simulink model "W02_B_three_ways"  (R2024b)
settings: Solver=ode4  StartTime=0  StopTime=T_final  FixedStep=h  RelTol=1e-3
values from neighbouring files (symbols this model uses):
  F_step = 1    [W02_0_setup.m]
  pid_b = 2    [W02_0_setup.m]
  pid_k = 2    [W02_0_setup.m]
  pid_m = 1    [W02_0_setup.m]
  t_step = 1    [W02_0_setup.m]
  x0_pos = 0    [W02_0_setup.m]    (also in W02_1_build_pid.m = 0.5 and Run: A and C swing back from 0.5 m,',    'B stays at)
  x0_vel = 0    [W02_0_setup.m]
settings Model: Creator=admin  LastModifiedBy=admin
settings DataIOCC: ReturnWorkspaceOutputs=off

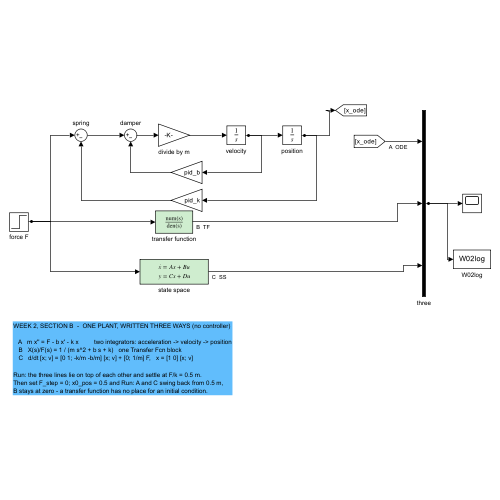
[thumbnail: Simulink's stored preview of the top-level diagram]
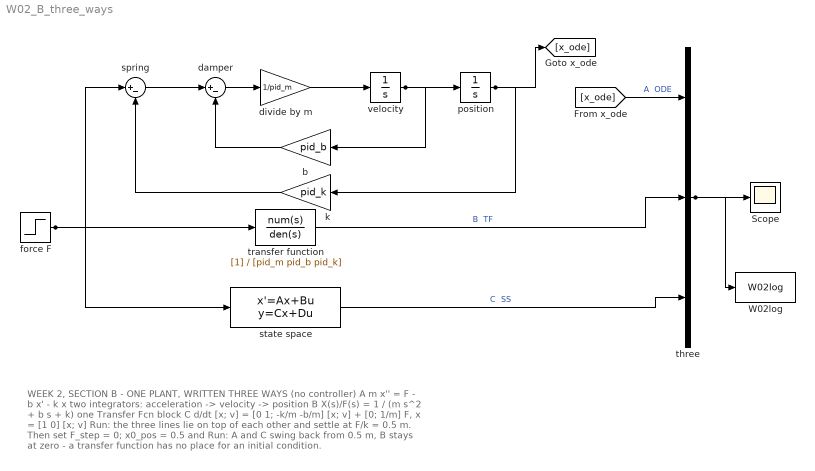
== system W02_B_three_ways ==
  note: WEEK 2, SECTION B  -  ONE PLANT, WRITTEN THREE WAYS (no controller)
      |
      |    A   m x'' = F - b x' - k x         two integrators: acceleration -> velocity -> position
      |    B   X(s)/F(s) = 1 / (m s^2 + b s + k)   one Transfer Fcn block
      |    C   d/dt [x; v] = [0 1; -k/m -b/m] [x; v] + [0; 1/m] F,   x = [1 0] [x; v]
      |
      | Run: the three lines lie on top of each other and settle at F/k = 0.5 m.
      | Then set F_step = 0; x0_pos = 0.5 and Run: A and C swing back from 0.5 m,
      | B stays at zero - a transfer function has no place for an initial condition.
  Scope : Scope
  W02log : ToWorkspace  VariableName=W02log  SaveFormat=Structure With Time  SampleTime=-1
  b : Gain  Gain=pid_b
  damper : Sum  Inputs=|+-
  divide by m : Gain  Gain=1/pid_m
  force F : Step  Time=t_step  After=F_step  SampleTime=0
  k : Gain  Gain=pid_k
  position : Integrator  InitialCondition=x0_pos
  spring : Sum  Inputs=|+-
  state space : StateSpace  A=[0 1; -pid_k/pid_m -pid_b/pid_m]  B=[0; 1/pid_m]  C=[1 0]  D=0  InitialCondition=[x0_pos; x0_vel]
  three : Mux  Inputs=3
  transfer function : TransferFcn  Denominator=[pid_m pid_b pid_k]
  velocity : Integrator  InitialCondition=x0_vel
  wires:
  force F/1 -> spring/1, transfer function/1, state space/1
  spring/1 -> damper/1
  damper/1 -> divide by m/1
  divide by m/1 -> velocity/1
  velocity/1 -> position/1, b/1
  b/1 -> damper/2
  position/1 -> k/1, [x_ode]
  k/1 -> spring/2
  [x_ode] -> three/1  "A  ODE"
  transfer function/1 -> three/2  "B  TF"
  state space/1 -> three/3  "C  SS"
  three/1 -> Scope/1, W02log/1
